simulink model "simiam_demo"  (Simulink 8.3)
settings: Solver=FixedStepDiscrete  StartTime=0.0  StopTime=Inf  FixedStep=0.033  RelTol=1e-3
undefined symbols (not defined in the file): magnitude
libraries: simiam x6, vrlib x2, simulink x1
settings Model: Creator=jdelacroix  LastModifiedBy=mcorberan
settings OptimizationCC: ExpressionDepthLimit=2147483647
settings DebuggingCC: FcnCallInpInsideContextMsg=EnableAllAsWarning
settings GRTTargetCC: CombineOutputUpdateFcns=on  GRTInterface=off

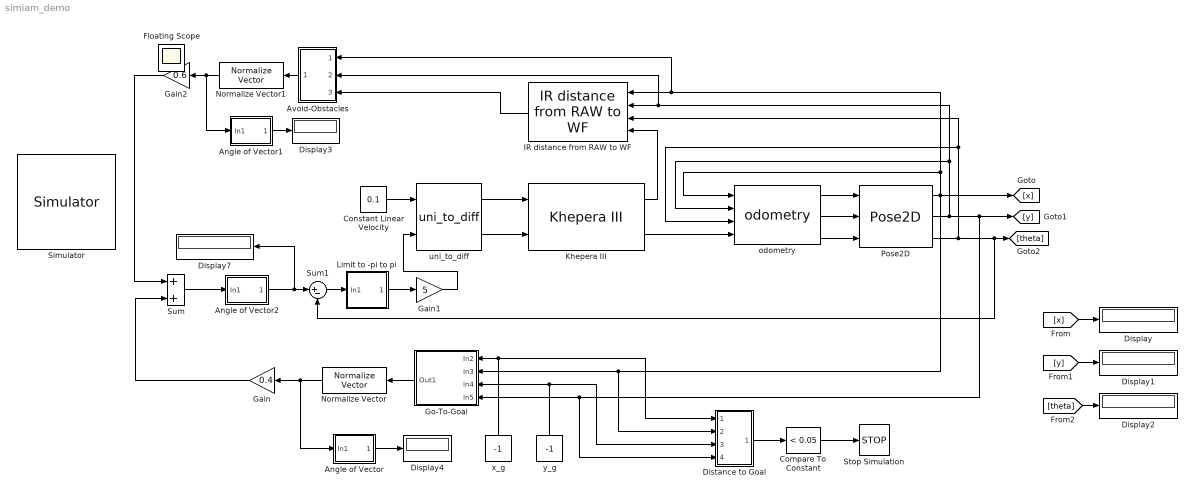
== system simiam_demo ==
  Angle of Vector : Subsystem
      mask Display:
      | port_label('input', 1, 'u')
      | port_label('output', 1, 'theta')
  Angle of Vector1 : Subsystem
      mask Display:
      | port_label('input', 1, 'u')
      | port_label('output', 1, 'theta')
  Angle of Vector2 : Subsystem
      mask Display:
      | port_label('input', 1, 'u')
      | port_label('output', 1, 'theta')
  Avoid-Obstacles : Subsystem
      mask Display:
      | port_label('input', 1, 'x')
      | port_label('input', 2, 'y')
      | port_label('input', 3, 'ir_wf')
      | port_label('output', 1, 'u_ao')
  Compare To Constant : simulink/Logic and Bit Operations/Compare To Constant  relop=<  const=0.05  OutDataTypeStr=boolean
  Constant Linear Velocity : Constant  Value=0.1
  Display{,1..4,7} (6 alike) : Display
  Distance to Goal : Subsystem
      mask Display:
      | port_label('input', 1, 'x_g')
      | port_label('input', 2, 'x')
      | port_label('input', 3, 'y_g')
      | port_label('input', 4, 'y')
      | port_label('output', 1, 'd')
  Gain : Gain  Gain=0.4
  Gain1 : Gain  Gain=5
  Gain2 : Gain  Gain=0.6
  Go-To-Goal : Subsystem
      mask Display:
      | port_label('input', 1, 'x_g')
      | port_label('input', 2, 'x')
      | port_label('input', 3, 'y_g')
      | port_label('input', 4, 'y')
      | port_label('output', 1, 'u_gtg')
  IR distance from RAW to WF : simiam/IR distance from RAW to WF
  Khepera III : simiam/Khepera III  x_0=0  y_0=0  theta_0=0  robot_id=1
  Limit to -pi to pi : Subsystem
      mask Display:
      | port_label('input', 1, 'e')
      | port_label('output', 1, 'e')
  Normalize Vector : vrlib/Utilities/Normalize Vector  maxzero=0
  Normalize Vector1 : vrlib/Utilities/Normalize Vector  maxzero=0
  Pose2D : simiam/Pose2D  SystemSampleTime=-1
  Simulator : simiam/Simulator  Priority=1
  Stop Simulation : Stop
  Sum : Sum
  Sum1 : Sum  Inputs=|+-
  odometry : simiam/odometry  wheel_radius=0.021  wheel_base_length=0.0885  ticks_per_rev=2675
  uni_to_diff : simiam/uni_to_diff  wheel_radius=0.021  wheel_base_length=0.0885
  x_g : Constant  Value=-1
  y_g : Constant  Value=-1
  Floating Scope : Scope
      settings: Floating=on
  wires:
  uni_to_diff/1 -> Khepera III/1
  uni_to_diff/2 -> Khepera III/2
  Constant Linear Velocity/1 -> uni_to_diff/1
  odometry/3 -> Pose2D/3
  odometry/2 -> Pose2D/2
  odometry/1 -> Pose2D/1
  Khepera III/2 -> odometry/4
  Pose2D/1 -> [x], odometry/1, Avoid-Obstacles/1(In1), IR distance from RAW to WF/1, Distance to Goal/2(In2), Go-To-Goal/2(In3)
  Pose2D/2 -> [y], Distance to Goal/4(In4), Go-To-Goal/4(In5), odometry/2, Avoid-Obstacles/2(In2), IR distance from RAW to WF/2
  [theta] -> Display2/1
  [y] -> Display1/1
  [x] -> Display/1
  x_g/1 -> Distance to Goal/1(In1), Go-To-Goal/1(In2)
  y_g/1 -> Distance to Goal/3(In3), Go-To-Goal/3(In4)
  Khepera III/1 -> IR distance from RAW to WF/4
  IR distance from RAW to WF/1 -> Avoid-Obstacles/3(In3)
  Avoid-Obstacles/1(Out1) -> Normalize Vector1/1
  Go-To-Goal/1(Out1) -> Normalize Vector/1
  Gain2/1 -> Sum/1
  Gain/1 -> Sum/2
  Sum1/1 -> Limit to -pi to pi/1(In1)
  Angle of Vector2/1(Out1) -> Display7/1, Sum1/1
  Pose2D/3 -> Sum1/2, [theta], IR distance from RAW to WF/3, odometry/3
  Gain1/1 -> uni_to_diff/2
  Limit to -pi to pi/1(Out1) -> Gain1/1
  Normalize Vector/1 -> Angle of Vector/1(In1), Gain/1
  Angle of Vector/1(Out1) -> Display4/1
  Normalize Vector1/1 -> Angle of Vector1/1(In1), Gain2/1
  Angle of Vector1/1(Out1) -> Display3/1
  Sum/1 -> Angle of Vector2/1(In1)
  Distance to Goal/1(Out1) -> Compare To Constant/1
  Compare To Constant/1 -> Stop Simulation/1

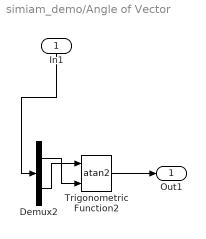
== system simiam_demo/Angle of Vector ==
  In1 : Inport
  Demux2 : Demux  Outputs=2
  Trigonometric Function2 : Trigonometry  Operator=atan2
  Out1 : Outport
  wires:
  Trigonometric Function2/1 -> Out1/1
  Demux2/1 -> Trigonometric Function2/2
  Demux2/2 -> Trigonometric Function2/1
  In1/1 -> Demux2/1

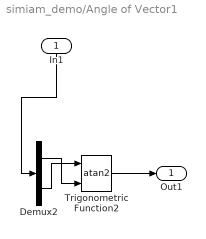
== system simiam_demo/Angle of Vector1 ==
  In1 : Inport
  Demux2 : Demux  Outputs=2
  Trigonometric Function2 : Trigonometry  Operator=atan2
  Out1 : Outport
  wires:
  Trigonometric Function2/1 -> Out1/1
  Demux2/1 -> Trigonometric Function2/2
  Demux2/2 -> Trigonometric Function2/1
  In1/1 -> Demux2/1

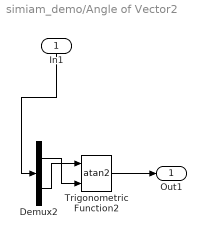
== system simiam_demo/Angle of Vector2 ==
  In1 : Inport
  Demux2 : Demux  Outputs=2
  Trigonometric Function2 : Trigonometry  Operator=atan2
  Out1 : Outport
  wires:
  Trigonometric Function2/1 -> Out1/1
  Demux2/1 -> Trigonometric Function2/2
  Demux2/2 -> Trigonometric Function2/1
  In1/1 -> Demux2/1

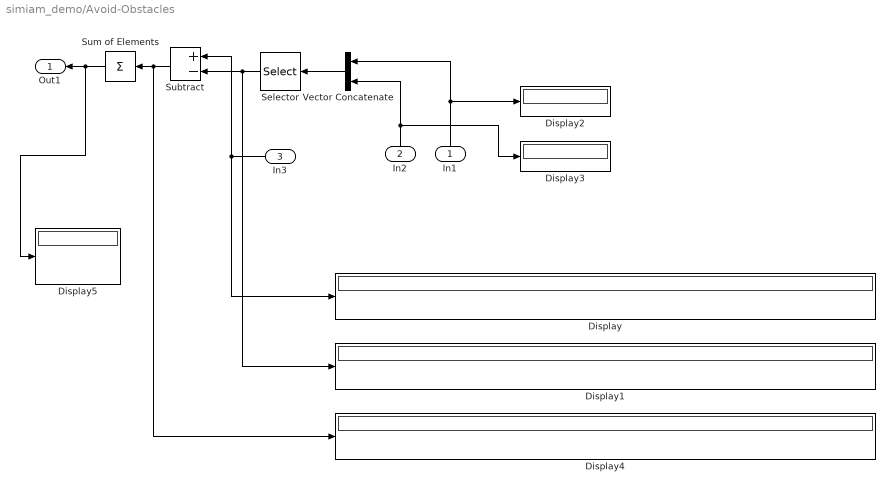
== system simiam_demo/Avoid-Obstacles ==
  In1 : Inport
  In2 : Inport  Port=2
  In3 : Inport  Port=3
  Display{,1..5} (6 alike) : Display
  Selector : Selector  NumberOfDimensions=2  IndexMode=Zero-based  InputPortWidth=3  IndexOptions=Select all,Index vector (dialog)  Indices=-1,[0 0 0 0 0 0 0 0 0]  OutputSizes=1,1
  Subtract : Sum  Inputs=+-
  Sum of Elements : Sum  Inputs=+  CollapseMode=Specified dimension  CollapseDim=2
  Vector Concatenate : Concatenate  Mode=Multidimensional array
  Out1 : Outport
  wires:
  Vector Concatenate/1 -> Selector/1
  Subtract/1 -> Display4/1, Sum of Elements/1
  Sum of Elements/1 -> Display5/1, Out1/1
  In3/1 -> Display/1, Subtract/1
  Selector/1 -> Display1/1, Subtract/2
  In1/1 -> Display2/1, Vector Concatenate/1
  In2/1 -> Display3/1, Vector Concatenate/2

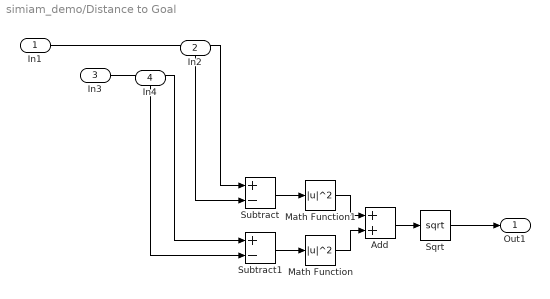
== system simiam_demo/Distance to Goal ==
  In1 : Inport
  In2 : Inport  Port=2
  In3 : Inport  Port=3
  In4 : Inport  Port=4
  Add : Sum
  Math Function : Math  Operator=magnitude^2  SaturateOnIntegerOverflow=on
  Math Function1 : Math  Operator=magnitude^2  SaturateOnIntegerOverflow=on
  Sqrt : Sqrt  SaturateOnIntegerOverflow=on
  Subtract : Sum  Inputs=+-
  Subtract1 : Sum  Inputs=+-
  Out1 : Outport
  wires:
  In4/1 -> Subtract1/2
  Subtract1/1 -> Math Function/1
  Math Function/1 -> Add/2
  Sqrt/1 -> Out1/1
  Subtract/1 -> Math Function1/1
  Math Function1/1 -> Add/1
  Add/1 -> Sqrt/1
  In2/1 -> Subtract/2
  In3/1 -> Subtract1/1
  In1/1 -> Subtract/1

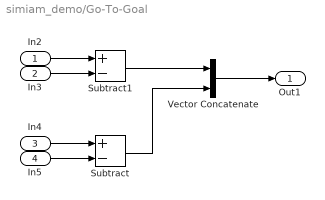
== system simiam_demo/Go-To-Goal ==
  In2 : Inport
  In3 : Inport  Port=2
  In4 : Inport  Port=3
  In5 : Inport  Port=4
  Subtract : Sum  Inputs=+-
  Subtract1 : Sum  Inputs=+-
  Vector Concatenate : Concatenate  Mode=Multidimensional array
  Out1 : Outport
  wires:
  In5/1 -> Subtract/2
  In2/1 -> Subtract1/1
  In3/1 -> Subtract1/2
  In4/1 -> Subtract/1
  Vector Concatenate/1 -> Out1/1
  Subtract1/1 -> Vector Concatenate/1
  Subtract/1 -> Vector Concatenate/2

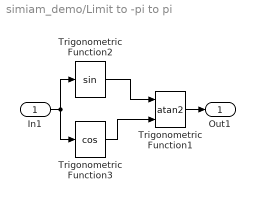
== system simiam_demo/Limit to -pi to pi ==
  In1 : Inport
  Trigonometric Function1 : Trigonometry  Operator=atan2
  Trigonometric Function2 : Trigonometry
  Trigonometric Function3 : Trigonometry  Operator=cos
  Out1 : Outport
  wires:
  In1/1 -> Trigonometric Function2/1, Trigonometric Function3/1
  Trigonometric Function3/1 -> Trigonometric Function1/2
  Trigonometric Function1/1 -> Out1/1
  Trigonometric Function2/1 -> Trigonometric Function1/1
